simulink model "gm_IP_Core_SS_Switch_and_PWM"  (R2021a)
settings: Solver=VariableStepAuto  StartTime=0.0  StopTime=0.001  RelTol=1e-3
undefined symbols (not defined in the file or in its folder): f_FPGA_clk, T_FPGA_clk
libraries: hdlmdlgenlib x3, hdlsllib x3, simulink x2
(part 2 of 3)

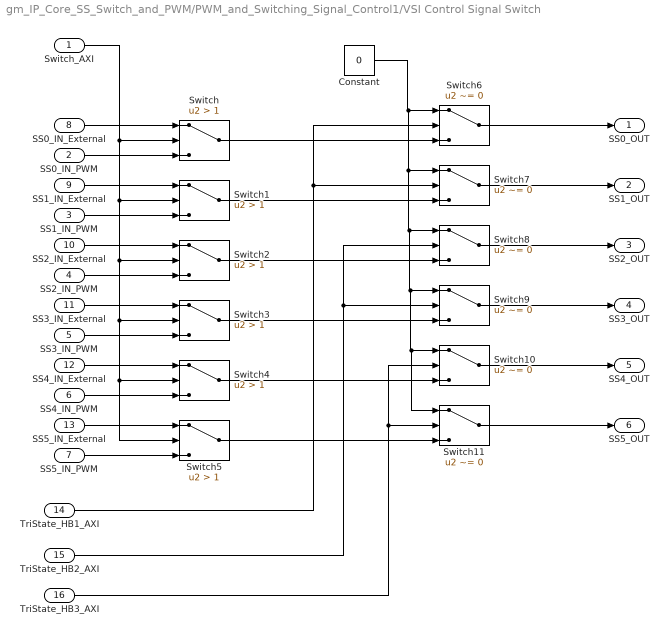
== system gm_IP_Core_SS_Switch_and_PWM/PWM_and_Switching_Signal_Control1/VSI Control Signal Switch ==
  Switch_AXI : Inport
  SS0_IN_PWM : Inport  Port=2
  SS1_IN_PWM : Inport  Port=3
  SS2_IN_PWM : Inport  Port=4
  SS3_IN_PWM : Inport  Port=5
  SS4_IN_PWM : Inport  Port=6
  SS5_IN_PWM : Inport  Port=7
  SS0_IN_External : Inport  Port=8
  SS1_IN_External : Inport  Port=9
  SS2_IN_External : Inport  Port=10
  SS3_IN_External : Inport  Port=11
  SS4_IN_External : Inport  Port=12
  SS5_IN_External : Inport  Port=13
  TriState_HB1_AXI : Inport  Port=14
  TriState_HB2_AXI : Inport  Port=15
  TriState_HB3_AXI : Inport  Port=16
  Constant : Constant  Value=0  OutDataTypeStr=boolean  SampleTime=T_FPGA_clk
  Switch{,1..5} (6 alike) : Switch  Criteria=u2 > Threshold  Threshold=1
  Switch{6..11} (6 alike) : Switch  Criteria=u2 ~= 0  Threshold=1
  SS0_OUT : Outport  VectorParamsAs1DForOutWhenUnconnected=off
  SS1_OUT : Outport  Port=2  VectorParamsAs1DForOutWhenUnconnected=off
  SS2_OUT : Outport  Port=3  VectorParamsAs1DForOutWhenUnconnected=off
  SS3_OUT : Outport  Port=4  VectorParamsAs1DForOutWhenUnconnected=off
  SS4_OUT : Outport  Port=5  VectorParamsAs1DForOutWhenUnconnected=off
  SS5_OUT : Outport  Port=6  VectorParamsAs1DForOutWhenUnconnected=off
  wires:
  Constant/1 -> Switch6/1, Switch7/1, Switch8/1, Switch9/1, Switch10/1, Switch11/1
  Switch6/1 -> SS0_OUT/1
  Switch7/1 -> SS1_OUT/1
  Switch8/1 -> SS2_OUT/1
  Switch9/1 -> SS3_OUT/1
  Switch10/1 -> SS4_OUT/1
  Switch11/1 -> SS5_OUT/1
  TriState_HB1_AXI/1 -> Switch7/2, Switch6/2
  TriState_HB2_AXI/1 -> Switch9/2, Switch8/2
  TriState_HB3_AXI/1 -> Switch11/2, Switch10/2
  SS5_IN_PWM/1 -> Switch5/3
  SS5_IN_External/1 -> Switch5/1
  SS4_IN_PWM/1 -> Switch4/3
  SS4_IN_External/1 -> Switch4/1
  SS3_IN_PWM/1 -> Switch3/3
  SS3_IN_External/1 -> Switch3/1
  SS2_IN_PWM/1 -> Switch2/3
  SS2_IN_External/1 -> Switch2/1
  SS1_IN_PWM/1 -> Switch1/3
  SS1_IN_External/1 -> Switch1/1
  SS0_IN_External/1 -> Switch/1
  SS0_IN_PWM/1 -> Switch/3
  Switch4/1 -> Switch10/3
  Switch1/1 -> Switch7/3
  Switch2/1 -> Switch8/3
  Switch3/1 -> Switch9/3
  Switch/1 -> Switch6/3
  Switch5/1 -> Switch11/3
  Switch_AXI/1 -> Switch/2, Switch1/2, Switch2/2, Switch3/2, Switch5/2, Switch4/2

== system gm_IP_Core_SS_Switch_and_PWM/PWM_and_Switching_Signal_Control/GenPWM/Counter Ctrl ==
  note: scaling triangle amplitude to 100
  hdl_cnt : Inport  OutDataTypeStr=fixdt(0, 20, 0)  PortDimensions=1  SampleTime=1e-08
  f_carrier_kHz : Inport  Port=2  OutDataTypeStr=fixdt(0, 25, 26)  PortDimensions=1  SampleTime=1e-08
  T_carrier_us : Inport  Port=3  OutDataTypeStr=fixdt(0, 25, 0)  PortDimensions=1  SampleTime=1e-08
  Constant1 : Constant  Value=0  OutDataTypeStr=fixdt(0, 20, 0)  SampleTime=1e-08
  Constant11 : Constant  Value=0  OutDataTypeStr=fixdt(0, 20, 0)  SampleTime=1e-08
  Constant12 : Constant  Value=0  OutDataTypeStr=boolean  SampleTime=1e-08
  Constant14 : Constant  OutDataTypeStr=boolean  SampleTime=1e-08
  Delay : Delay  DelayLength=double(1)  InitialCondition=0  SampleTime=1e-08
  Delay6 : Delay  DelayLength=double(1)  InitialCondition=0  SampleTime=1e-08
  Logical Operator : Logic  Operator=OR  AllPortsSameDT=off  OutDataTypeStr=boolean  SampleTime=1e-08
  Product : Product  Inputs=**  OutDataTypeStr=fixdt(0, 18, 17)  SampleTime=1e-08
  Relational Operator1 : RelationalOperator  Operator===  OutDataTypeStr=boolean  SampleTime=1e-08  RndMeth=Nearest
  Relational Operator2 : RelationalOperator  Operator===  OutDataTypeStr=boolean  SampleTime=1e-08  RndMeth=Nearest
  Relational Operator4 : RelationalOperator  OutDataTypeStr=boolean  SampleTime=1e-08  RndMeth=Nearest
  Relational Operator5 : RelationalOperator  Operator=<=  OutDataTypeStr=boolean  SampleTime=1e-08  RndMeth=Nearest
  Switch6 : Switch  Criteria=u2 > Threshold  Threshold=double(0)  OutDataTypeStr=boolean  SampleTime=1e-08
  Switch7 : Switch  Criteria=u2 > Threshold  Threshold=double(0)  OutDataTypeStr=boolean  SampleTime=1e-08
  dir_ctrl : Outport  SampleTime=1e-08  VectorParamsAs1DForOutWhenUnconnected=off
  triangle_sig : Outport  Port=2  SampleTime=1e-08  VectorParamsAs1DForOutWhenUnconnected=off
  Period_CenterMax : Outport  Port=3  SampleTime=1e-08  VectorParamsAs1DForOutWhenUnconnected=off
  Period_CenterMin : Outport  Port=4  SampleTime=1e-08  VectorParamsAs1DForOutWhenUnconnected=off
  wires:
  hdl_cnt/1 -> Relational Operator5/1, Relational Operator4/1, Relational Operator2/1, Relational Operator1/1, Product/1
  f_carrier_kHz/1 -> Delay/1
  T_carrier_us/1 -> Relational Operator4/2, Relational Operator1/2
  Constant1/1 -> Relational Operator2/2
  Constant11/1 -> Relational Operator5/2
  Constant12/1 -> Switch7/1
  Constant14/1 -> Switch7/3
  Delay/1 -> Product/2
  Delay6/1 -> Switch6/3
  Logical Operator/1 -> Switch6/2
  Product/1 -> triangle_sig/1
  Relational Operator1/1 -> Period_CenterMax/1
  Relational Operator2/1 -> Period_CenterMin/1
  Relational Operator4/1 -> Switch7/2, Logical Operator/1
  Relational Operator5/1 -> Logical Operator/2
  Switch6/1 -> Delay6/1, dir_ctrl/1
  Switch7/1 -> Switch6/1

== system gm_IP_Core_SS_Switch_and_PWM/PWM_and_Switching_Signal_Control/GenPWM/LimitPulseWidth ==
  note: Set pulse width between 0-1
  ref_sig : Inport  OutDataTypeStr=fixdt(1, 14, 12)  PortDimensions=1  SampleTime=1e-08
  min_pulse_width : Inport  Port=2  OutDataTypeStr=fixdt(1, 18, 16)  PortDimensions=1  SampleTime=1e-08
  Add : Sum  Inputs=+-  AccumDataTypeStr=fixdt(1, 19, 16)  OutDataTypeStr=fixdt(1, 18, 16)  SampleTime=1e-08
  Constant : Constant  OutDataTypeStr=fixdt(1, 18, 16)  SampleTime=1e-08
  Constant1 : Constant  Value=1.0099945068359375  OutDataTypeStr=fixdt(1, 18, 16)  SampleTime=1e-08
  Constant2 : Constant  Value=0  OutDataTypeStr=fixdt(1, 18, 16)  SampleTime=1e-08
  Logical Operator : Logic  Operator=OR  AllPortsSameDT=off  OutDataTypeStr=boolean  SampleTime=1e-08
  Relational Operator : RelationalOperator  Operator=>  OutDataTypeStr=boolean  SampleTime=1e-08  RndMeth=Nearest
  Relational Operator1 : RelationalOperator  Operator=<  OutDataTypeStr=boolean  SampleTime=1e-08  RndMeth=Nearest
  Saturation : Saturate  UpperLimit="fi(0,1,18,16,\"hex\",\"10000\")"  LowerLimit="fi(0,1,18,16,\"hex\",\"00000\")"  SampleTime=1e-08  OutDataTypeStr=fixdt(1, 18, 16)
  Switch1 : Switch  Criteria=u2 > Threshold  Threshold=double(0)  OutDataTypeStr=fixdt(1, 18, 16)  SampleTime=1e-08
  Switch6 : Switch  Criteria=u2 > Threshold  Threshold=double(0)  OutDataTypeStr=fixdt(1, 18, 16)  SampleTime=1e-08
  ref_sig_limit : Outport  SampleTime=1e-08  VectorParamsAs1DForOutWhenUnconnected=off
  wires:
  Add/1 -> Relational Operator/2
  Constant/1 -> Add/1
  Constant1/1 -> Switch1/3
  Constant2/1 -> Switch1/1
  Logical Operator/1 -> Switch6/2
  Relational Operator/1 -> Logical Operator/1
  Relational Operator1/1 -> Switch1/2, Logical Operator/2
  Saturation/1 -> Relational Operator1/2
  Switch1/1 -> Switch6/1
  Switch6/1 -> ref_sig_limit/1
  ref_sig/1 -> Switch6/3, Relational Operator1/1, Relational Operator/1
  min_pulse_width/1 -> Saturation/1, Add/2

== system gm_IP_Core_SS_Switch_and_PWM/PWM_and_Switching_Signal_Control/GenPWM/LimitPulseWidth1 ==
  note: Set pulse width in percent
  ref_sig : Inport  OutDataTypeStr=fixdt(1, 14, 12)  PortDimensions=1  SampleTime=1e-08
  min_pulse_width : Inport  Port=2  OutDataTypeStr=fixdt(1, 18, 16)  PortDimensions=1  SampleTime=1e-08
  Add : Sum  Inputs=+-  AccumDataTypeStr=fixdt(1, 19, 16)  OutDataTypeStr=fixdt(1, 18, 16)  SampleTime=1e-08
  Constant : Constant  OutDataTypeStr=fixdt(1, 18, 16)  SampleTime=1e-08
  Constant1 : Constant  Value=1.0099945068359375  OutDataTypeStr=fixdt(1, 18, 16)  SampleTime=1e-08
  Constant2 : Constant  Value=0  OutDataTypeStr=fixdt(1, 18, 16)  SampleTime=1e-08
  Logical Operator : Logic  Operator=OR  AllPortsSameDT=off  OutDataTypeStr=boolean  SampleTime=1e-08
  Relational Operator : RelationalOperator  Operator=>  OutDataTypeStr=boolean  SampleTime=1e-08  RndMeth=Nearest
  Relational Operator1 : RelationalOperator  Operator=<  OutDataTypeStr=boolean  SampleTime=1e-08  RndMeth=Nearest
  Saturation : Saturate  UpperLimit="fi(0,1,18,16,\"hex\",\"10000\")"  LowerLimit="fi(0,1,18,16,\"hex\",\"00000\")"  SampleTime=1e-08  OutDataTypeStr=fixdt(1, 18, 16)
  Switch1 : Switch  Criteria=u2 > Threshold  Threshold=double(0)  OutDataTypeStr=fixdt(1, 18, 16)  SampleTime=1e-08
  Switch6 : Switch  Criteria=u2 > Threshold  Threshold=double(0)  OutDataTypeStr=fixdt(1, 18, 16)  SampleTime=1e-08
  ref_sig_limit : Outport  SampleTime=1e-08  VectorParamsAs1DForOutWhenUnconnected=off
  wires:
  Add/1 -> Relational Operator/2
  Constant/1 -> Add/1
  Constant1/1 -> Switch1/3
  Constant2/1 -> Switch1/1
  Logical Operator/1 -> Switch6/2
  Relational Operator/1 -> Logical Operator/1
  Relational Operator1/1 -> Switch1/2, Logical Operator/2
  Saturation/1 -> Relational Operator1/2
  Switch1/1 -> Switch6/1
  Switch6/1 -> ref_sig_limit/1
  ref_sig/1 -> Switch6/3, Relational Operator1/1, Relational Operator/1
  min_pulse_width/1 -> Saturation/1, Add/2

== system gm_IP_Core_SS_Switch_and_PWM/PWM_and_Switching_Signal_Control/GenPWM/LimitPulseWidth2 ==
  note: Set pulse width in percent
  ref_sig : Inport  OutDataTypeStr=fixdt(1, 14, 12)  PortDimensions=1  SampleTime=1e-08
  min_pulse_width : Inport  Port=2  OutDataTypeStr=fixdt(1, 18, 16)  PortDimensions=1  SampleTime=1e-08
  Add : Sum  Inputs=+-  AccumDataTypeStr=fixdt(1, 19, 16)  OutDataTypeStr=fixdt(1, 18, 16)  SampleTime=1e-08
  Constant : Constant  OutDataTypeStr=fixdt(1, 18, 16)  SampleTime=1e-08
  Constant1 : Constant  Value=1.0099945068359375  OutDataTypeStr=fixdt(1, 18, 16)  SampleTime=1e-08
  Constant2 : Constant  Value=0  OutDataTypeStr=fixdt(1, 18, 16)  SampleTime=1e-08
  Logical Operator : Logic  Operator=OR  AllPortsSameDT=off  OutDataTypeStr=boolean  SampleTime=1e-08
  Relational Operator : RelationalOperator  Operator=>  OutDataTypeStr=boolean  SampleTime=1e-08  RndMeth=Nearest
  Relational Operator1 : RelationalOperator  Operator=<  OutDataTypeStr=boolean  SampleTime=1e-08  RndMeth=Nearest
  Saturation : Saturate  UpperLimit="fi(0,1,18,16,\"hex\",\"10000\")"  LowerLimit="fi(0,1,18,16,\"hex\",\"00000\")"  SampleTime=1e-08  OutDataTypeStr=fixdt(1, 18, 16)
  Switch1 : Switch  Criteria=u2 > Threshold  Threshold=double(0)  OutDataTypeStr=fixdt(1, 18, 16)  SampleTime=1e-08
  Switch6 : Switch  Criteria=u2 > Threshold  Threshold=double(0)  OutDataTypeStr=fixdt(1, 18, 16)  SampleTime=1e-08
  ref_sig_limit : Outport  SampleTime=1e-08  VectorParamsAs1DForOutWhenUnconnected=off
  wires:
  Add/1 -> Relational Operator/2
  Constant/1 -> Add/1
  Constant1/1 -> Switch1/3
  Constant2/1 -> Switch1/1
  Logical Operator/1 -> Switch6/2
  Relational Operator/1 -> Logical Operator/1
  Relational Operator1/1 -> Switch1/2, Logical Operator/2
  Saturation/1 -> Relational Operator1/2
  Switch1/1 -> Switch6/1
  Switch6/1 -> ref_sig_limit/1
  ref_sig/1 -> Switch6/3, Relational Operator1/1, Relational Operator/1
  min_pulse_width/1 -> Saturation/1, Add/2

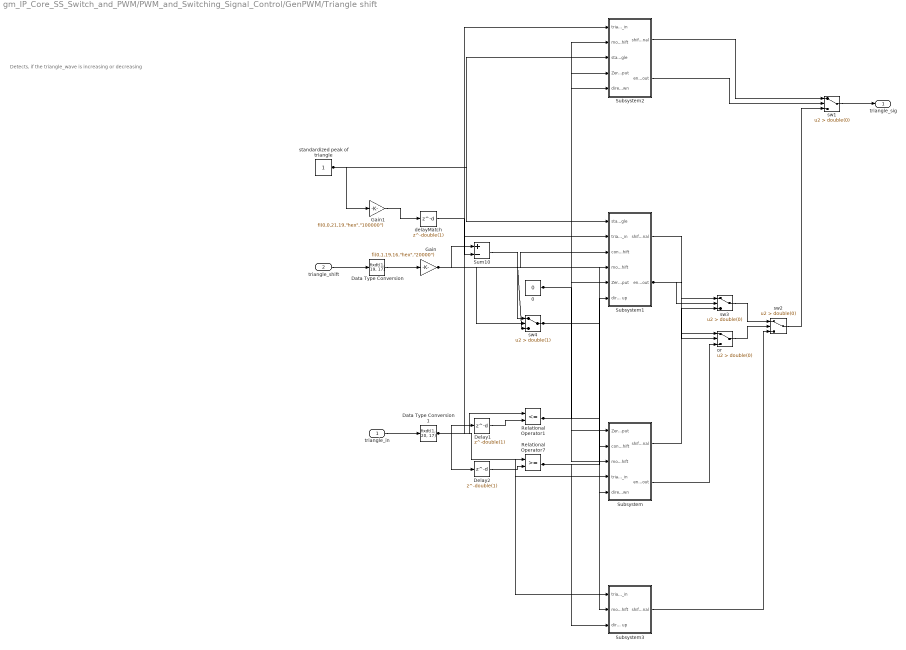
== system gm_IP_Core_SS_Switch_and_PWM/PWM_and_Switching_Signal_Control/GenPWM/Triangle shift ==
  note: Detects, if the triangle_wave is increasing or decreasing
  triangle_in : Inport  OutDataTypeStr=fixdt(0, 18, 17)  PortDimensions=1  SampleTime=1e-08
  triangle_shift : Inport  Port=2  OutDataTypeStr=fixdt(0, 18, 17)  PortDimensions=1  SampleTime=1e-08
  0 : Constant  Value=0  OutDataTypeStr=boolean  SampleTime=1e-08
  Data Type Conversion : DataTypeConversion  OutDataTypeStr=fixdt(1, 19, 17)  SampleTime=1e-08
  Data Type Conversion1 : DataTypeConversion  OutDataTypeStr=fixdt(1, 20, 17)  SampleTime=1e-08
  Delay1 : Delay  DelayLength=double(1)  InitialCondition=0  SampleTime=1e-08
  Delay2 : Delay  DelayLength=double(1)  InitialCondition=0  SampleTime=1e-08
  Gain : Gain  Gain="fi(0,1,19,16,\"hex\",\"20000\")"  ParamDataTypeStr=fixdt(1, 19, 16)  OutDataTypeStr=fixdt(1, 20, 17)  SampleTime=1e-08
  Gain1 : Gain  Gain="fi(0,0,21,19,\"hex\",\"100000\")"  ParamDataTypeStr=fixdt(0, 21, 19)  OutDataTypeStr=fixdt(1, 20, 17)  SampleTime=1e-08
  Relational Operator1 : RelationalOperator  Operator=<=  OutDataTypeStr=boolean  SampleTime=1e-08  RndMeth=Nearest
  Relational Operator7 : RelationalOperator  OutDataTypeStr=boolean  SampleTime=1e-08  RndMeth=Nearest
  Subsystem : Subsystem
  Subsystem1 : Subsystem
  Subsystem2 : Subsystem
  Subsystem3 : Subsystem
  Sum10 : Sum  Inputs=+-  AccumDataTypeStr=fixdt(1, 21, 17)  OutDataTypeStr=fixdt(1, 20, 17)  SampleTime=1e-08
  delayMatch : Delay  DelayLength=double(1)  InitialCondition=0  SampleTime=1e-08
  or : Switch  Criteria=u2 > Threshold  Threshold=double(0)  OutDataTypeStr=boolean  SampleTime=1e-08
  standardized peak of triangle : Constant  OutDataTypeStr=fixdt(0, 21, 17)  SampleTime=1e-08
  sw1 : Switch  Criteria=u2 > Threshold  Threshold=double(0)  OutDataTypeStr=fixdt(1, 18, 16)  SampleTime=1e-08
  sw2 : Switch  Criteria=u2 > Threshold  Threshold=double(0)  OutDataTypeStr=fixdt(1, 21, 17)  SampleTime=1e-08
  sw3 : Switch  Criteria=u2 > Threshold  Threshold=double(0)  OutDataTypeStr=fixdt(1, 21, 17)  SampleTime=1e-08
  sw4 : Switch  Criteria=u2 > Threshold  Threshold=double(1)  OutDataTypeStr=fixdt(1, 20, 17)  SampleTime=1e-08
  triangle_sig : Outport  SampleTime=1e-08  VectorParamsAs1DForOutWhenUnconnected=off
  wires:
  0/1 -> Subsystem2/4(Zero_input), Subsystem1/5(Zero_input), Subsystem/1(Zero_input)
  Data Type Conversion/1 -> Gain/1
  Data Type Conversion1/1 -> Relational Operator7/1, Relational Operator1/1, Delay2/1, Delay1/1, Subsystem3/1(triangle_in), Subsystem2/1(triangle_in), Subsystem/4(triangle_in), Subsystem1/2(triangle_in)
  Delay1/1 -> Relational Operator1/2
  Delay2/1 -> Relational Operator7/2
  Gain/1 -> sw4/3, sw4/2, Sum10/1, Subsystem/2(converted triangle_shift), Subsystem1/3(converted triangle_shift)
  delayMatch/1 -> Sum10/2
  Relational Operator1/1 -> Subsystem/5(direction down), Subsystem2/5(direction down)
  Relational Operator7/1 -> Subsystem1/6(direction up), Subsystem3/3(direction up)
  Subsystem/1(shifted triangle_in signal) -> sw3/3
  Subsystem/2(enable_out) -> or/3
  Subsystem1/1(shifted triangle_in signal) -> sw3/1
  Subsystem1/2(enable_out) -> sw3/2, or/2, or/1
  Subsystem2/1(shifted triangle_in signal) -> sw1/1
  Subsystem2/2(enable_out) -> sw1/2
  Subsystem3/1(shifted triangle_in signal) -> sw2/3
  Sum10/1 -> sw4/1
  or/1 -> sw2/2
  standardized peak of triangle/1 -> Gain1/1, Subsystem2/3(standardized peak of triangle), Subsystem1/1(standardized peak of triangle)
  sw1/1 -> triangle_sig/1
  sw2/1 -> sw1/3
  sw3/1 -> sw2/1
  sw4/1 -> Subsystem3/2(modified triangle_shift), Subsystem/3(modified triangle_shift), Subsystem1/4(modified triangle_shift), Subsystem2/2(modified triangle_shift)
  triangle_in/1 -> Data Type Conversion1/1
  triangle_shift/1 -> Data Type Conversion/1
  Gain1/1 -> delayMatch/1

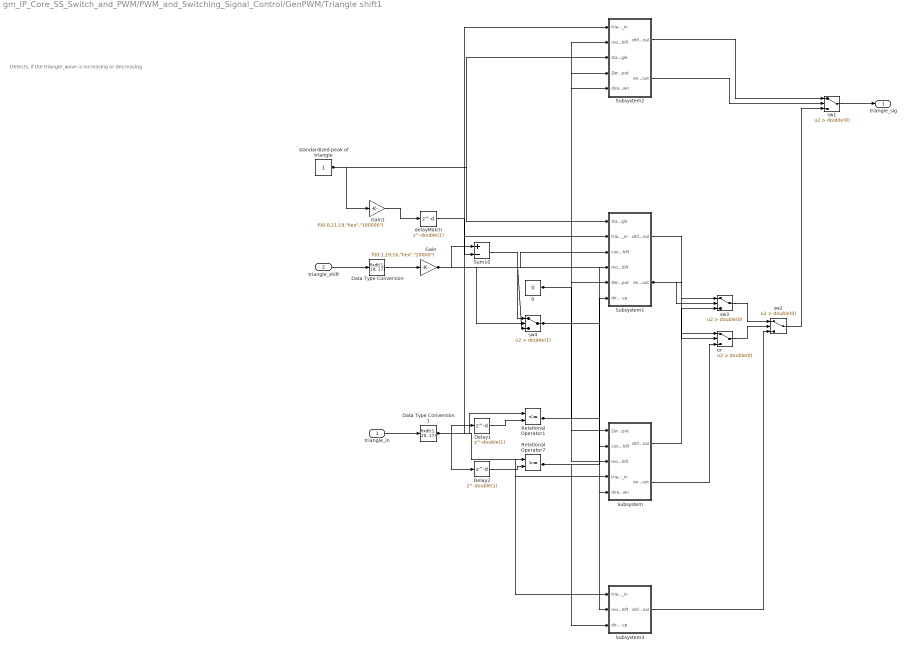
== system gm_IP_Core_SS_Switch_and_PWM/PWM_and_Switching_Signal_Control/GenPWM/Triangle shift1 ==
  note: Detects, if the triangle_wave is increasing or decreasing
  triangle_in : Inport  OutDataTypeStr=fixdt(0, 18, 17)  PortDimensions=1  SampleTime=1e-08
  triangle_shift : Inport  Port=2  OutDataTypeStr=fixdt(0, 18, 17)  PortDimensions=1  SampleTime=1e-08
  0 : Constant  Value=0  OutDataTypeStr=boolean  SampleTime=1e-08
  Data Type Conversion : DataTypeConversion  OutDataTypeStr=fixdt(1, 19, 17)  SampleTime=1e-08
  Data Type Conversion1 : DataTypeConversion  OutDataTypeStr=fixdt(1, 20, 17)  SampleTime=1e-08
  Delay1 : Delay  DelayLength=double(1)  InitialCondition=0  SampleTime=1e-08
  Delay2 : Delay  DelayLength=double(1)  InitialCondition=0  SampleTime=1e-08
  Gain : Gain  Gain="fi(0,1,19,16,\"hex\",\"20000\")"  ParamDataTypeStr=fixdt(1, 19, 16)  OutDataTypeStr=fixdt(1, 20, 17)  SampleTime=1e-08
  Gain1 : Gain  Gain="fi(0,0,21,19,\"hex\",\"100000\")"  ParamDataTypeStr=fixdt(0, 21, 19)  OutDataTypeStr=fixdt(1, 20, 17)  SampleTime=1e-08
  Relational Operator1 : RelationalOperator  Operator=<=  OutDataTypeStr=boolean  SampleTime=1e-08  RndMeth=Nearest
  Relational Operator7 : RelationalOperator  OutDataTypeStr=boolean  SampleTime=1e-08  RndMeth=Nearest
  Subsystem : Subsystem
  Subsystem1 : Subsystem
  Subsystem2 : Subsystem
  Subsystem3 : Subsystem
  Sum10 : Sum  Inputs=+-  AccumDataTypeStr=fixdt(1, 21, 17)  OutDataTypeStr=fixdt(1, 20, 17)  SampleTime=1e-08
  delayMatch : Delay  DelayLength=double(1)  InitialCondition=0  SampleTime=1e-08
  or : Switch  Criteria=u2 > Threshold  Threshold=double(0)  OutDataTypeStr=boolean  SampleTime=1e-08
  standardized peak of triangle : Constant  OutDataTypeStr=fixdt(0, 21, 17)  SampleTime=1e-08
  sw1 : Switch  Criteria=u2 > Threshold  Threshold=double(0)  OutDataTypeStr=fixdt(1, 18, 16)  SampleTime=1e-08
  sw2 : Switch  Criteria=u2 > Threshold  Threshold=double(0)  OutDataTypeStr=fixdt(1, 21, 17)  SampleTime=1e-08
  sw3 : Switch  Criteria=u2 > Threshold  Threshold=double(0)  OutDataTypeStr=fixdt(1, 21, 17)  SampleTime=1e-08
  sw4 : Switch  Criteria=u2 > Threshold  Threshold=double(1)  OutDataTypeStr=fixdt(1, 20, 17)  SampleTime=1e-08
  triangle_sig : Outport  SampleTime=1e-08  VectorParamsAs1DForOutWhenUnconnected=off
  wires:
  0/1 -> Subsystem2/4(Zero_input), Subsystem1/5(Zero_input), Subsystem/1(Zero_input)
  Data Type Conversion/1 -> Gain/1
  Data Type Conversion1/1 -> Relational Operator7/1, Relational Operator1/1, Delay2/1, Delay1/1, Subsystem3/1(triangle_in), Subsystem2/1(triangle_in), Subsystem/4(triangle_in), Subsystem1/2(triangle_in)
  Delay1/1 -> Relational Operator1/2
  Delay2/1 -> Relational Operator7/2
  Gain/1 -> sw4/3, sw4/2, Sum10/1, Subsystem/2(converted triangle_shift), Subsystem1/3(converted triangle_shift)
  delayMatch/1 -> Sum10/2
  Relational Operator1/1 -> Subsystem/5(direction down), Subsystem2/5(direction down)
  Relational Operator7/1 -> Subsystem1/6(direction up), Subsystem3/3(direction up)
  Subsystem/1(shifted triangle_in signal) -> sw3/3
  Subsystem/2(enable_out) -> or/3
  Subsystem1/1(shifted triangle_in signal) -> sw3/1
  Subsystem1/2(enable_out) -> sw3/2, or/2, or/1
  Subsystem2/1(shifted triangle_in signal) -> sw1/1
  Subsystem2/2(enable_out) -> sw1/2
  Subsystem3/1(shifted triangle_in signal) -> sw2/3
  Sum10/1 -> sw4/1
  or/1 -> sw2/2
  standardized peak of triangle/1 -> Gain1/1, Subsystem2/3(standardized peak of triangle), Subsystem1/1(standardized peak of triangle)
  sw1/1 -> triangle_sig/1
  sw2/1 -> sw1/3
  sw3/1 -> sw2/1
  sw4/1 -> Subsystem3/2(modified triangle_shift), Subsystem/3(modified triangle_shift), Subsystem1/4(modified triangle_shift), Subsystem2/2(modified triangle_shift)
  triangle_in/1 -> Data Type Conversion1/1
  triangle_shift/1 -> Data Type Conversion/1
  Gain1/1 -> delayMatch/1

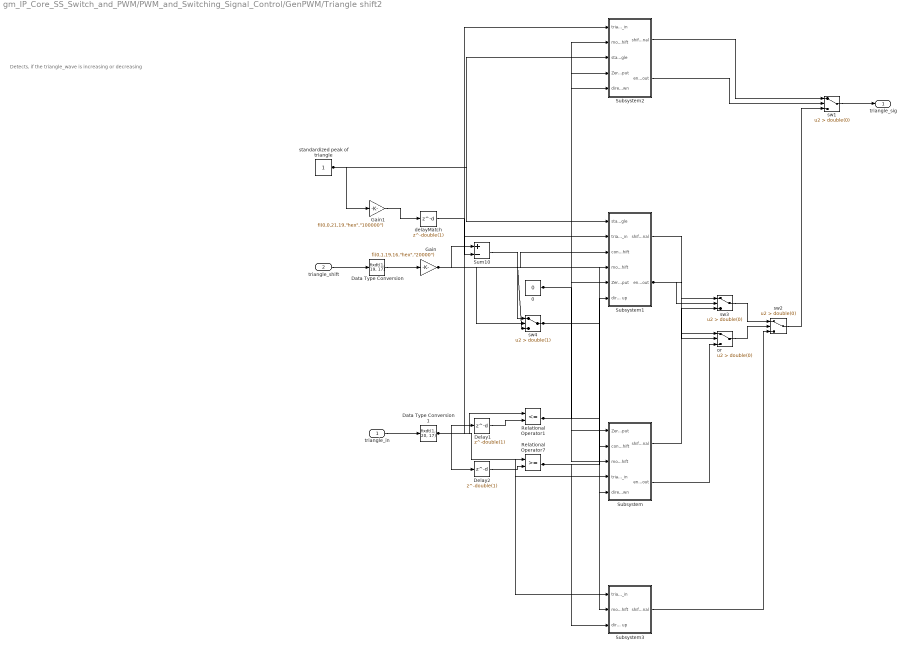
== system gm_IP_Core_SS_Switch_and_PWM/PWM_and_Switching_Signal_Control/GenPWM/Triangle shift2 ==
  note: Detects, if the triangle_wave is increasing or decreasing
  triangle_in : Inport  OutDataTypeStr=fixdt(0, 18, 17)  PortDimensions=1  SampleTime=1e-08
  triangle_shift : Inport  Port=2  OutDataTypeStr=fixdt(0, 18, 17)  PortDimensions=1  SampleTime=1e-08
  0 : Constant  Value=0  OutDataTypeStr=boolean  SampleTime=1e-08
  Data Type Conversion : DataTypeConversion  OutDataTypeStr=fixdt(1, 19, 17)  SampleTime=1e-08
  Data Type Conversion1 : DataTypeConversion  OutDataTypeStr=fixdt(1, 20, 17)  SampleTime=1e-08
  Delay1 : Delay  DelayLength=double(1)  InitialCondition=0  SampleTime=1e-08
  Delay2 : Delay  DelayLength=double(1)  InitialCondition=0  SampleTime=1e-08
  Gain : Gain  Gain="fi(0,1,19,16,\"hex\",\"20000\")"  ParamDataTypeStr=fixdt(1, 19, 16)  OutDataTypeStr=fixdt(1, 20, 17)  SampleTime=1e-08
  Gain1 : Gain  Gain="fi(0,0,21,19,\"hex\",\"100000\")"  ParamDataTypeStr=fixdt(0, 21, 19)  OutDataTypeStr=fixdt(1, 20, 17)  SampleTime=1e-08
  Relational Operator1 : RelationalOperator  Operator=<=  OutDataTypeStr=boolean  SampleTime=1e-08  RndMeth=Nearest
  Relational Operator7 : RelationalOperator  OutDataTypeStr=boolean  SampleTime=1e-08  RndMeth=Nearest
  Subsystem : Subsystem
  Subsystem1 : Subsystem
  Subsystem2 : Subsystem
  Subsystem3 : Subsystem
  Sum10 : Sum  Inputs=+-  AccumDataTypeStr=fixdt(1, 21, 17)  OutDataTypeStr=fixdt(1, 20, 17)  SampleTime=1e-08
  delayMatch : Delay  DelayLength=double(1)  InitialCondition=0  SampleTime=1e-08
  or : Switch  Criteria=u2 > Threshold  Threshold=double(0)  OutDataTypeStr=boolean  SampleTime=1e-08
  standardized peak of triangle : Constant  OutDataTypeStr=fixdt(0, 21, 17)  SampleTime=1e-08
  sw1 : Switch  Criteria=u2 > Threshold  Threshold=double(0)  OutDataTypeStr=fixdt(1, 18, 16)  SampleTime=1e-08
  sw2 : Switch  Criteria=u2 > Threshold  Threshold=double(0)  OutDataTypeStr=fixdt(1, 21, 17)  SampleTime=1e-08
  sw3 : Switch  Criteria=u2 > Threshold  Threshold=double(0)  OutDataTypeStr=fixdt(1, 21, 17)  SampleTime=1e-08
  sw4 : Switch  Criteria=u2 > Threshold  Threshold=double(1)  OutDataTypeStr=fixdt(1, 20, 17)  SampleTime=1e-08
  triangle_sig : Outport  SampleTime=1e-08  VectorParamsAs1DForOutWhenUnconnected=off
  wires:
  0/1 -> Subsystem2/4(Zero_input), Subsystem1/5(Zero_input), Subsystem/1(Zero_input)
  Data Type Conversion/1 -> Gain/1
  Data Type Conversion1/1 -> Relational Operator7/1, Relational Operator1/1, Delay2/1, Delay1/1, Subsystem3/1(triangle_in), Subsystem2/1(triangle_in), Subsystem/4(triangle_in), Subsystem1/2(triangle_in)
  Delay1/1 -> Relational Operator1/2
  Delay2/1 -> Relational Operator7/2
  Gain/1 -> sw4/3, sw4/2, Sum10/1, Subsystem/2(converted triangle_shift), Subsystem1/3(converted triangle_shift)
  delayMatch/1 -> Sum10/2
  Relational Operator1/1 -> Subsystem/5(direction down), Subsystem2/5(direction down)
  Relational Operator7/1 -> Subsystem1/6(direction up), Subsystem3/3(direction up)
  Subsystem/1(shifted triangle_in signal) -> sw3/3
  Subsystem/2(enable_out) -> or/3
  Subsystem1/1(shifted triangle_in signal) -> sw3/1
  Subsystem1/2(enable_out) -> sw3/2, or/2, or/1
  Subsystem2/1(shifted triangle_in signal) -> sw1/1
  Subsystem2/2(enable_out) -> sw1/2
  Subsystem3/1(shifted triangle_in signal) -> sw2/3
  Sum10/1 -> sw4/1
  or/1 -> sw2/2
  standardized peak of triangle/1 -> Gain1/1, Subsystem2/3(standardized peak of triangle), Subsystem1/1(standardized peak of triangle)
  sw1/1 -> triangle_sig/1
  sw2/1 -> sw1/3
  sw3/1 -> sw2/1
  sw4/1 -> Subsystem3/2(modified triangle_shift), Subsystem/3(modified triangle_shift), Subsystem1/4(modified triangle_shift), Subsystem2/2(modified triangle_shift)
  triangle_in/1 -> Data Type Conversion1/1
  triangle_shift/1 -> Data Type Conversion/1
  Gain1/1 -> delayMatch/1

== system gm_IP_Core_SS_Switch_and_PWM/PWM_and_Switching_Signal_Control1/GenPWM/Counter Ctrl ==
  note: scaling triangle amplitude to 100
  note: if (hdl_cnt >= step_cnt)
      | 	dir_ctrl = true;
      | else if (hdl_cnt <= 0)
      | 	dir_ctrl = false;
      | else
      | 	dir_ctrl = dir_ctrl;
  hdl_cnt : Inport
  f_carrier_kHz : Inport  Port=2
  T_carrier_us : Inport  Port=3
  Constant1 : Constant  Value=0  OutDataTypeStr=fixdt(0,20,0)  SampleTime=T_FPGA_clk
  Constant11 : Constant  Value=0  OutDataTypeStr=fixdt(0,20,0)  SampleTime=T_FPGA_clk
  Constant12 : Constant  Value=false  SampleTime=T_FPGA_clk
  Constant14 : Constant  Value=true  SampleTime=T_FPGA_clk
  Delay : Delay  DelayLength=1
  Delay6 : Delay  DelayLength=1
  Logical Operator : Logic  Operator=OR  AllPortsSameDT=off  OutDataTypeStr=boolean
  Product : Product  OutDataTypeStr=fixdt(0,18,17)
  Relational Operator1 : RelationalOperator  Operator===  OutDataTypeStr=boolean  RndMeth=Nearest
  Relational Operator2 : RelationalOperator  Operator===  OutDataTypeStr=boolean  RndMeth=Nearest
  Relational Operator4 : RelationalOperator  OutDataTypeStr=boolean  RndMeth=Nearest
  Relational Operator5 : RelationalOperator  Operator=<=  OutDataTypeStr=boolean  RndMeth=Nearest
  Scope9 : Scope  NumInputPorts=2
  Switch6 : Switch  Criteria=u2 > Threshold
  Switch7 : Switch  Criteria=u2 > Threshold
  dir_ctrl : Outport  VectorParamsAs1DForOutWhenUnconnected=off
  triangle_sig : Outport  Port=2  VectorParamsAs1DForOutWhenUnconnected=off
  Period_CenterMax : Outport  Port=3  VectorParamsAs1DForOutWhenUnconnected=off
  Period_CenterMin : Outport  Port=4  VectorParamsAs1DForOutWhenUnconnected=off
  wires:
  Product/1 -> triangle_sig/1
  Constant1/1 -> Relational Operator2/2
  Relational Operator2/1 -> Period_CenterMin/1
  Relational Operator1/1 -> Period_CenterMax/1
  Delay/1 -> Product/2, Scope9/2
  f_carrier_kHz/1 -> Delay/1
  T_carrier_us/1 -> Relational Operator1/2, Relational Operator4/2
  Delay6/1 -> Switch6/3
  Constant14/1 -> Switch7/3
  Constant12/1 -> Switch7/1
  Switch7/1 -> Switch6/1
  Logical Operator/1 -> Switch6/2
  Constant11/1 -> Relational Operator5/2
  Relational Operator5/1 -> Logical Operator/2
  Relational Operator4/1 -> Logical Operator/1, Switch7/2
  Switch6/1 -> dir_ctrl/1, Delay6/1
  hdl_cnt/1 -> Scope9/1, Product/1, Relational Operator4/1, Relational Operator5/1, Relational Operator1/1, Relational Operator2/1

== system gm_IP_Core_SS_Switch_and_PWM/PWM_and_Switching_Signal_Control1/GenPWM/LimitPulseWidth ==
  note: Set pulse width between 0-1
  ref_sig : Inport
  min_pulse_width : Inport  Port=2
  Add : Sum  Inputs=+-  OutDataTypeStr=Inherit: Same as first input
  Constant : Constant  OutDataTypeStr=fixdt(1,18,16)  SampleTime=T_FPGA_clk
  Constant1 : Constant  Value=1.01  OutDataTypeStr=fixdt(1,18,16)  SampleTime=T_FPGA_clk
  Constant2 : Constant  Value=0  OutDataTypeStr=fixdt(1,18,16)  SampleTime=T_FPGA_clk
  Logical Operator : Logic  Operator=OR  AllPortsSameDT=off  OutDataTypeStr=boolean
  Relational Operator : RelationalOperator  Operator=>  OutDataTypeStr=boolean  RndMeth=Nearest
  Relational Operator1 : RelationalOperator  Operator=<  OutDataTypeStr=boolean  RndMeth=Nearest
  Saturation : Saturate  UpperLimit=1  LowerLimit=0  OutDataTypeStr=fixdt(1,18,16)
  Switch1 : Switch  Criteria=u2 > Threshold
  Switch6 : Switch  Criteria=u2 > Threshold
  ref_sig_limit : Outport  VectorParamsAs1DForOutWhenUnconnected=off
  wires:
  Saturation/1 -> Relational Operator1/2
  Switch6/1 -> ref_sig_limit/1
  Constant2/1 -> Switch1/1
  Switch1/1 -> Switch6/1
  Constant1/1 -> Switch1/3
  Logical Operator/1 -> Switch6/2
  Relational Operator1/1 -> Switch1/2, Logical Operator/2
  Relational Operator/1 -> Logical Operator/1
  ref_sig/1 -> Relational Operator1/1, Relational Operator/1, Switch6/3
  Add/1 -> Relational Operator/2
  min_pulse_width/1 -> Saturation/1, Add/2
  Constant/1 -> Add/1

== system gm_IP_Core_SS_Switch_and_PWM/PWM_and_Switching_Signal_Control1/GenPWM/LimitPulseWidth1 ==
  note: Set pulse width in percent
  ref_sig : Inport
  min_pulse_width : Inport  Port=2
  Add : Sum  Inputs=+-  OutDataTypeStr=Inherit: Same as first input
  Constant : Constant  OutDataTypeStr=fixdt(1,18,16)  SampleTime=T_FPGA_clk
  Constant1 : Constant  Value=1.01  OutDataTypeStr=fixdt(1,18,16)  SampleTime=T_FPGA_clk
  Constant2 : Constant  Value=0  OutDataTypeStr=fixdt(1,18,16)  SampleTime=T_FPGA_clk
  Logical Operator : Logic  Operator=OR  AllPortsSameDT=off  OutDataTypeStr=boolean
  Relational Operator : RelationalOperator  Operator=>  OutDataTypeStr=boolean  RndMeth=Nearest
  Relational Operator1 : RelationalOperator  Operator=<  OutDataTypeStr=boolean  RndMeth=Nearest
  Saturation : Saturate  UpperLimit=1  LowerLimit=0  OutDataTypeStr=fixdt(1,18,16)
  Switch1 : Switch  Criteria=u2 > Threshold
  Switch6 : Switch  Criteria=u2 > Threshold
  ref_sig_limit : Outport  VectorParamsAs1DForOutWhenUnconnected=off
  wires:
  Saturation/1 -> Relational Operator1/2
  Switch6/1 -> ref_sig_limit/1
  Constant2/1 -> Switch1/1
  Switch1/1 -> Switch6/1
  Constant1/1 -> Switch1/3
  Logical Operator/1 -> Switch6/2
  Relational Operator1/1 -> Switch1/2, Logical Operator/2
  Relational Operator/1 -> Logical Operator/1
  ref_sig/1 -> Relational Operator1/1, Relational Operator/1, Switch6/3
  Add/1 -> Relational Operator/2
  min_pulse_width/1 -> Saturation/1, Add/2
  Constant/1 -> Add/1

== system gm_IP_Core_SS_Switch_and_PWM/PWM_and_Switching_Signal_Control1/GenPWM/LimitPulseWidth2 ==
  note: Set pulse width in percent
  ref_sig : Inport
  min_pulse_width : Inport  Port=2
  Add : Sum  Inputs=+-  OutDataTypeStr=Inherit: Same as first input
  Constant : Constant  OutDataTypeStr=fixdt(1,18,16)  SampleTime=T_FPGA_clk
  Constant1 : Constant  Value=1.01  OutDataTypeStr=fixdt(1,18,16)  SampleTime=T_FPGA_clk
  Constant2 : Constant  Value=0  OutDataTypeStr=fixdt(1,18,16)  SampleTime=T_FPGA_clk
  Logical Operator : Logic  Operator=OR  AllPortsSameDT=off  OutDataTypeStr=boolean
  Relational Operator : RelationalOperator  Operator=>  OutDataTypeStr=boolean  RndMeth=Nearest
  Relational Operator1 : RelationalOperator  Operator=<  OutDataTypeStr=boolean  RndMeth=Nearest
  Saturation : Saturate  UpperLimit=1  LowerLimit=0  OutDataTypeStr=fixdt(1,18,16)
  Switch1 : Switch  Criteria=u2 > Threshold
  Switch6 : Switch  Criteria=u2 > Threshold
  ref_sig_limit : Outport  VectorParamsAs1DForOutWhenUnconnected=off
  wires:
  Saturation/1 -> Relational Operator1/2
  Switch6/1 -> ref_sig_limit/1
  Constant2/1 -> Switch1/1
  Switch1/1 -> Switch6/1
  Constant1/1 -> Switch1/3
  Logical Operator/1 -> Switch6/2
  Relational Operator1/1 -> Switch1/2, Logical Operator/2
  Relational Operator/1 -> Logical Operator/1
  ref_sig/1 -> Relational Operator1/1, Relational Operator/1, Switch6/3
  Add/1 -> Relational Operator/2
  min_pulse_width/1 -> Saturation/1, Add/2
  Constant/1 -> Add/1

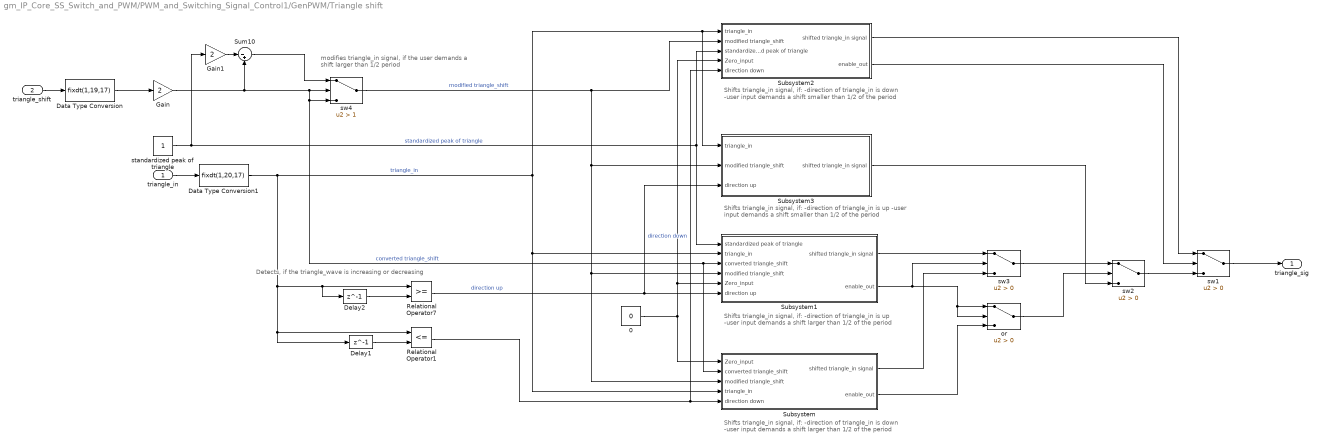
== system gm_IP_Core_SS_Switch_and_PWM/PWM_and_Switching_Signal_Control1/GenPWM/Triangle shift ==
  note: Shifts triangle_in signal, if:
      | -direction of triangle_in is down
      | -user input demands a shift smaller than 1/2 of the period
  note: Shifts triangle_in signal, if:
      | -direction of triangle_in is up
      | -user input demands a shift smaller than 1/2 of the period
  note: Shifts triangle_in signal, if:
      | -direction of triangle_in is up
      | -user input demands a shift larger than 1/2 of the period
  note: Shifts triangle_in signal, if:
      | -direction of triangle_in is down
      | -user input demands a shift larger than 1/2 of the period
  note: Detects, if the triangle_wave is increasing or decreasing
  note: modifies triangle_in signal,
      | if the user demands a shift larger than 1/2 period
  triangle_in : Inport
  triangle_shift : Inport  Port=2
  0 : Constant  Value=0  OutDataTypeStr=boolean  SampleTime=T_FPGA_clk
  Data Type Conversion : DataTypeConversion  OutDataTypeStr=fixdt(1,19,17)
  Data Type Conversion1 : DataTypeConversion  OutDataTypeStr=fixdt(1,20,17)
  Delay1 : Delay  DelayLength=1
  Delay2 : Delay  DelayLength=1
  Gain : Gain  Gain=2  OutDataTypeStr=fixdt(1,20,17)
  Gain1 : Gain  Gain=2  OutDataTypeStr=fixdt(1,20,17)
  Relational Operator1 : RelationalOperator  Operator=<=  OutDataTypeStr=boolean  RndMeth=Nearest
  Relational Operator7 : RelationalOperator  OutDataTypeStr=boolean  RndMeth=Nearest
  Subsystem : Subsystem
  Subsystem1 : Subsystem
  Subsystem2 : Subsystem
  Subsystem3 : Subsystem
  Sum10 : Sum  Inputs=|-+  OutDataTypeStr=fixdt(1,20,17)
  or : Switch  Criteria=u2 > Threshold
  standardized peak of triangle : Constant  OutDataTypeStr=fixdt(0,21,17)  SampleTime=T_FPGA_clk
  sw1 : Switch  Criteria=u2 > Threshold  OutDataTypeStr=fixdt(1,18,16)
  sw2 : Switch  Criteria=u2 > Threshold
  sw3 : Switch  Criteria=u2 > Threshold
  sw4 : Switch  Criteria=u2 > Threshold  Threshold=1  OutDataTypeStr=fixdt(1,20,17)
  triangle_sig : Outport  VectorParamsAs1DForOutWhenUnconnected=off
  wires:
  Subsystem3/1(shifted triangle_in signal) -> sw2/3
  Subsystem2/2(enable_out) -> sw1/2
  Subsystem2/1(shifted triangle_in signal) -> sw1/1
  Subsystem1/1(shifted triangle_in signal) -> sw3/1
  Subsystem1/2(enable_out) -> sw3/2, or/1, or/2
  Subsystem/2(enable_out) -> or/3
  Subsystem/1(shifted triangle_in signal) -> sw3/3
  0/1 -> Subsystem/1(Zero_input), Subsystem1/5(Zero_input), Subsystem2/4(Zero_input)
  Delay1/1 -> Relational Operator1/2
  Relational Operator1/1 -> Subsystem2/5(direction down), Subsystem/5(direction down)  "direction down"
  triangle_in/1 -> Data Type Conversion1/1
  Data Type Conversion/1 -> Gain/1
  sw2/1 -> sw1/3
  Gain1/1 -> Sum10/1
  triangle_shift/1 -> Data Type Conversion/1
  standardized peak of triangle/1 -> Gain1/1, Subsystem1/1(standardized peak of triangle), Subsystem2/3(standardized peak of triangle)  "standardized peak of triangle"
  sw1/1 -> triangle_sig/1
  Sum10/1 -> sw4/1
  Gain/1 -> sw4/2, sw4/3, Subsystem1/3(converted triangle_shift), Subsystem/2(converted triangle_shift), Sum10/2  "converted triangle_shift"
  sw4/1 -> Subsystem2/2(modified triangle_shift), Subsystem1/4(modified triangle_shift), Subsystem/3(modified triangle_shift), Subsystem3/2(modified triangle_shift)  "modified triangle_shift"
  or/1 -> sw2/2
  Relational Operator7/1 -> Subsystem3/3(direction up), Subsystem1/6(direction up)  "direction up"
  sw3/1 -> sw2/1
  Data Type Conversion1/1 -> Relational Operator7/1, Delay2/1, Delay1/1, Relational Operator1/1, Subsystem1/2(triangle_in), Subsystem/4(triangle_in), Subsystem2/1(triangle_in), Subsystem3/1(triangle_in)  "triangle_in"
  Delay2/1 -> Relational Operator7/2

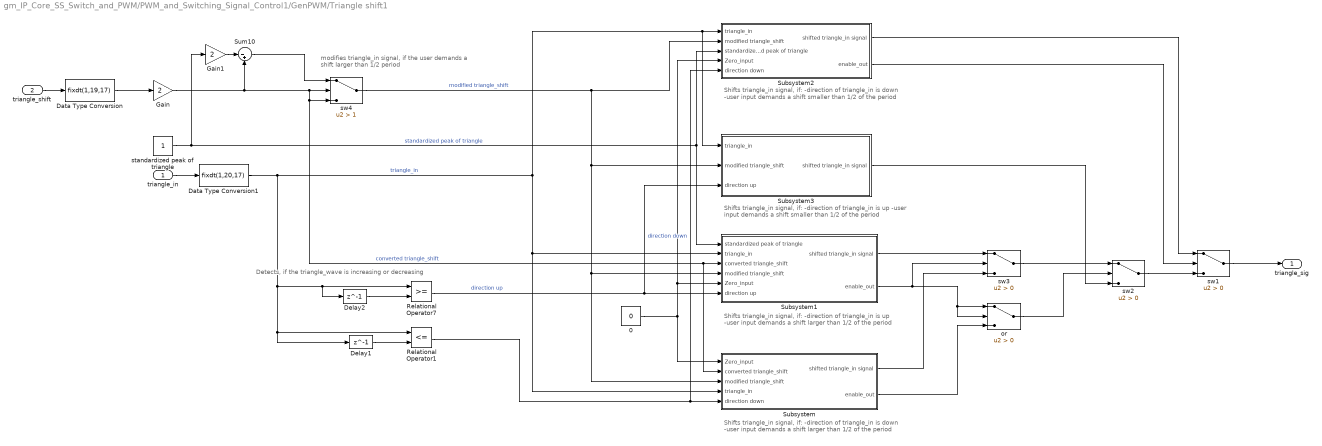
== system gm_IP_Core_SS_Switch_and_PWM/PWM_and_Switching_Signal_Control1/GenPWM/Triangle shift1 ==
  note: Shifts triangle_in signal, if:
      | -direction of triangle_in is down
      | -user input demands a shift smaller than 1/2 of the period
  note: Shifts triangle_in signal, if:
      | -direction of triangle_in is up
      | -user input demands a shift smaller than 1/2 of the period
  note: Shifts triangle_in signal, if:
      | -direction of triangle_in is up
      | -user input demands a shift larger than 1/2 of the period
  note: Shifts triangle_in signal, if:
      | -direction of triangle_in is down
      | -user input demands a shift larger than 1/2 of the period
  note: Detects, if the triangle_wave is increasing or decreasing
  note: modifies triangle_in signal,
      | if the user demands a shift larger than 1/2 period
  triangle_in : Inport
  triangle_shift : Inport  Port=2
  0 : Constant  Value=0  OutDataTypeStr=boolean  SampleTime=T_FPGA_clk
  Data Type Conversion : DataTypeConversion  OutDataTypeStr=fixdt(1,19,17)
  Data Type Conversion1 : DataTypeConversion  OutDataTypeStr=fixdt(1,20,17)
  Delay1 : Delay  DelayLength=1
  Delay2 : Delay  DelayLength=1
  Gain : Gain  Gain=2  OutDataTypeStr=fixdt(1,20,17)
  Gain1 : Gain  Gain=2  OutDataTypeStr=fixdt(1,20,17)
  Relational Operator1 : RelationalOperator  Operator=<=  OutDataTypeStr=boolean  RndMeth=Nearest
  Relational Operator7 : RelationalOperator  OutDataTypeStr=boolean  RndMeth=Nearest
  Subsystem : Subsystem
  Subsystem1 : Subsystem
  Subsystem2 : Subsystem
  Subsystem3 : Subsystem
  Sum10 : Sum  Inputs=|-+  OutDataTypeStr=fixdt(1,20,17)
  or : Switch  Criteria=u2 > Threshold
  standardized peak of triangle : Constant  OutDataTypeStr=fixdt(0,21,17)  SampleTime=T_FPGA_clk
  sw1 : Switch  Criteria=u2 > Threshold  OutDataTypeStr=fixdt(1,18,16)
  sw2 : Switch  Criteria=u2 > Threshold
  sw3 : Switch  Criteria=u2 > Threshold
  sw4 : Switch  Criteria=u2 > Threshold  Threshold=1  OutDataTypeStr=fixdt(1,20,17)
  triangle_sig : Outport  VectorParamsAs1DForOutWhenUnconnected=off
  wires:
  Subsystem3/1(shifted triangle_in signal) -> sw2/3
  Subsystem2/2(enable_out) -> sw1/2
  Subsystem2/1(shifted triangle_in signal) -> sw1/1
  Subsystem1/1(shifted triangle_in signal) -> sw3/1
  Subsystem1/2(enable_out) -> sw3/2, or/1, or/2
  Subsystem/2(enable_out) -> or/3
  Subsystem/1(shifted triangle_in signal) -> sw3/3
  0/1 -> Subsystem/1(Zero_input), Subsystem1/5(Zero_input), Subsystem2/4(Zero_input)
  Delay1/1 -> Relational Operator1/2
  Relational Operator1/1 -> Subsystem2/5(direction down), Subsystem/5(direction down)  "direction down"
  triangle_in/1 -> Data Type Conversion1/1
  Data Type Conversion/1 -> Gain/1
  sw2/1 -> sw1/3
  Gain1/1 -> Sum10/1
  triangle_shift/1 -> Data Type Conversion/1
  standardized peak of triangle/1 -> Gain1/1, Subsystem1/1(standardized peak of triangle), Subsystem2/3(standardized peak of triangle)  "standardized peak of triangle"
  sw1/1 -> triangle_sig/1
  Sum10/1 -> sw4/1
  Gain/1 -> sw4/2, sw4/3, Subsystem1/3(converted triangle_shift), Subsystem/2(converted triangle_shift), Sum10/2  "converted triangle_shift"
  sw4/1 -> Subsystem2/2(modified triangle_shift), Subsystem1/4(modified triangle_shift), Subsystem/3(modified triangle_shift), Subsystem3/2(modified triangle_shift)  "modified triangle_shift"
  or/1 -> sw2/2
  Relational Operator7/1 -> Subsystem3/3(direction up), Subsystem1/6(direction up)  "direction up"
  sw3/1 -> sw2/1
  Data Type Conversion1/1 -> Relational Operator7/1, Delay2/1, Delay1/1, Relational Operator1/1, Subsystem1/2(triangle_in), Subsystem/4(triangle_in), Subsystem2/1(triangle_in), Subsystem3/1(triangle_in)  "triangle_in"
  Delay2/1 -> Relational Operator7/2

== system gm_IP_Core_SS_Switch_and_PWM/PWM_and_Switching_Signal_Control1/GenPWM/Triangle shift2 ==
  note: Shifts triangle_in signal, if:
      | -direction of triangle_in is down
      | -user input demands a shift smaller than 1/2 of the period
  note: Shifts triangle_in signal, if:
      | -direction of triangle_in is up
      | -user input demands a shift smaller than 1/2 of the period
  note: Shifts triangle_in signal, if:
      | -direction of triangle_in is up
      | -user input demands a shift larger than 1/2 of the period
  note: Shifts triangle_in signal, if:
      | -direction of triangle_in is down
      | -user input demands a shift larger than 1/2 of the period
  note: Detects, if the triangle_wave is increasing or decreasing
  note: modifies triangle_in signal,
      | if the user demands a shift larger than 1/2 period
  triangle_in : Inport
  triangle_shift : Inport  Port=2
  0 : Constant  Value=0  OutDataTypeStr=boolean  SampleTime=T_FPGA_clk
  Data Type Conversion : DataTypeConversion  OutDataTypeStr=fixdt(1,19,17)
  Data Type Conversion1 : DataTypeConversion  OutDataTypeStr=fixdt(1,20,17)
  Delay1 : Delay  DelayLength=1
  Delay2 : Delay  DelayLength=1
  Gain : Gain  Gain=2  OutDataTypeStr=fixdt(1,20,17)
  Gain1 : Gain  Gain=2  OutDataTypeStr=fixdt(1,20,17)
  Relational Operator1 : RelationalOperator  Operator=<=  OutDataTypeStr=boolean  RndMeth=Nearest
  Relational Operator7 : RelationalOperator  OutDataTypeStr=boolean  RndMeth=Nearest
  Subsystem : Subsystem
  Subsystem1 : Subsystem
  Subsystem2 : Subsystem
  Subsystem3 : Subsystem
  Sum10 : Sum  Inputs=|-+  OutDataTypeStr=fixdt(1,20,17)
  or : Switch  Criteria=u2 > Threshold
  standardized peak of triangle : Constant  OutDataTypeStr=fixdt(0,21,17)  SampleTime=T_FPGA_clk
  sw1 : Switch  Criteria=u2 > Threshold  OutDataTypeStr=fixdt(1,18,16)
  sw2 : Switch  Criteria=u2 > Threshold
  sw3 : Switch  Criteria=u2 > Threshold
  sw4 : Switch  Criteria=u2 > Threshold  Threshold=1  OutDataTypeStr=fixdt(1,20,17)
  triangle_sig : Outport  VectorParamsAs1DForOutWhenUnconnected=off
  wires:
  Subsystem3/1(shifted triangle_in signal) -> sw2/3
  Subsystem2/2(enable_out) -> sw1/2
  Subsystem2/1(shifted triangle_in signal) -> sw1/1
  Subsystem1/1(shifted triangle_in signal) -> sw3/1
  Subsystem1/2(enable_out) -> sw3/2, or/1, or/2
  Subsystem/2(enable_out) -> or/3
  Subsystem/1(shifted triangle_in signal) -> sw3/3
  0/1 -> Subsystem/1(Zero_input), Subsystem1/5(Zero_input), Subsystem2/4(Zero_input)
  Delay1/1 -> Relational Operator1/2
  Relational Operator1/1 -> Subsystem2/5(direction down), Subsystem/5(direction down)  "direction down"
  triangle_in/1 -> Data Type Conversion1/1
  Data Type Conversion/1 -> Gain/1
  sw2/1 -> sw1/3
  Gain1/1 -> Sum10/1
  triangle_shift/1 -> Data Type Conversion/1
  standardized peak of triangle/1 -> Gain1/1, Subsystem1/1(standardized peak of triangle), Subsystem2/3(standardized peak of triangle)  "standardized peak of triangle"
  sw1/1 -> triangle_sig/1
  Sum10/1 -> sw4/1
  Gain/1 -> sw4/2, sw4/3, Subsystem1/3(converted triangle_shift), Subsystem/2(converted triangle_shift), Sum10/2  "converted triangle_shift"
  sw4/1 -> Subsystem2/2(modified triangle_shift), Subsystem1/4(modified triangle_shift), Subsystem/3(modified triangle_shift), Subsystem3/2(modified triangle_shift)  "modified triangle_shift"
  or/1 -> sw2/2
  Relational Operator7/1 -> Subsystem3/3(direction up), Subsystem1/6(direction up)  "direction up"
  sw3/1 -> sw2/1
  Data Type Conversion1/1 -> Relational Operator7/1, Delay2/1, Delay1/1, Relational Operator1/1, Subsystem1/2(triangle_in), Subsystem/4(triangle_in), Subsystem2/1(triangle_in), Subsystem3/1(triangle_in)  "triangle_in"
  Delay2/1 -> Relational Operator7/2

== system gm_IP_Core_SS_Switch_and_PWM/PWM_and_Switching_Signal_Control/GenPWM/Triangle shift/Subsystem ==
  Zero_input : Inport  OutDataTypeStr=boolean  PortDimensions=1  SampleTime=1e-08
  converted triangle_shift : Inport  Port=2  OutDataTypeStr=fixdt(1, 20, 17)  PortDimensions=1  SampleTime=1e-08
  modified triangle_shift : Inport  Port=3  OutDataTypeStr=fixdt(1, 20, 17)  PortDimensions=1  SampleTime=1e-08
  triangle_in : Inport  Port=4  OutDataTypeStr=fixdt(1, 20, 17)  PortDimensions=1  SampleTime=1e-08
  direction down : Inport  Port=5  OutDataTypeStr=boolean  PortDimensions=1  SampleTime=1e-08
  Relational Operator11 : RelationalOperator  Operator=<=  OutDataTypeStr=boolean  SampleTime=1e-08  RndMeth=Nearest
  Sum8 : Sum  Inputs=+-  AccumDataTypeStr=fixdt(1, 21, 17)  OutDataTypeStr=fixdt(1, 21, 17)  SampleTime=1e-08
  Unary Minus : UnaryMinus  SampleTime=1e-08
  and2_1 : Switch  Criteria=u2 > Threshold  Threshold=double(0)  OutDataTypeStr=boolean  SampleTime=1e-08
  and2_2 : Switch  Criteria=u2 > Threshold  Threshold=double(0)  OutDataTypeStr=boolean  SampleTime=1e-08
  delayMatch : Delay  DelayLength=double(1)  InitialCondition=0  SampleTime=1e-08
  delayMatch1 : Delay  DelayLength=double(1)  InitialCondition=0  SampleTime=1e-08
  shifted triangle_in signal : Outport  SampleTime=1e-08
  enable_out : Outport  Port=2  SampleTime=1e-08
  wires:
  delayMatch/1 -> and2_1/3
  Relational Operator11/1 -> and2_1/2
  Sum8/1 -> shifted triangle_in signal/1
  Unary Minus/1 -> Sum8/1, Relational Operator11/2
  and2_1/1 -> and2_2/1
  and2_2/1 -> enable_out/1
  Zero_input/1 -> delayMatch1/1, delayMatch/1
  converted triangle_shift/1 -> and2_1/1
  modified triangle_shift/1 -> Unary Minus/1
  triangle_in/1 -> Sum8/2, Relational Operator11/1
  direction down/1 -> and2_2/2
  delayMatch1/1 -> and2_2/3

== system gm_IP_Core_SS_Switch_and_PWM/PWM_and_Switching_Signal_Control/GenPWM/Triangle shift/Subsystem1 ==
  standardized peak of triangle : Inport  OutDataTypeStr=fixdt(0, 21, 17)  PortDimensions=1  SampleTime=1e-08
  triangle_in : Inport  Port=2  OutDataTypeStr=fixdt(1, 20, 17)  PortDimensions=1  SampleTime=1e-08
  converted triangle_shift : Inport  Port=3  OutDataTypeStr=fixdt(1, 20, 17)  PortDimensions=1  SampleTime=1e-08
  modified triangle_shift : Inport  Port=4  OutDataTypeStr=fixdt(1, 20, 17)  PortDimensions=1  SampleTime=1e-08
  Zero_input : Inport  Port=5  OutDataTypeStr=boolean  PortDimensions=1  SampleTime=1e-08
  direction up : Inport  Port=6  OutDataTypeStr=boolean  PortDimensions=1  SampleTime=1e-08
  Relational Operator2 : RelationalOperator  OutDataTypeStr=boolean  SampleTime=1e-08  RndMeth=Nearest
  Sum11_stage2 : Sum  AccumDataTypeStr=fixdt(1, 24, 17)  OutDataTypeStr=fixdt(1, 24, 17)  SampleTime=1e-08
  Sum11_stage3 : Sum  Inputs=+-  AccumDataTypeStr=fixdt(1, 24, 17)  OutDataTypeStr=fixdt(1, 21, 17)  SampleTime=1e-08
  Sum6 : Sum  AccumDataTypeStr=fixdt(1, 23, 17)  OutDataTypeStr=fixdt(1, 23, 17)  SampleTime=1e-08
  and1_1 : Switch  Criteria=u2 > Threshold  Threshold=double(0)  OutDataTypeStr=boolean  SampleTime=1e-08
  and1_2 : Switch  Criteria=u2 > Threshold  Threshold=double(0)  OutDataTypeStr=boolean  SampleTime=1e-08
  delayMatch{,1..3} (4 alike) : Delay  DelayLength=double(1)  InitialCondition=0  SampleTime=1e-08
  shifted triangle_in signal : Outport  SampleTime=1e-08
  enable_out : Outport  Port=2  SampleTime=1e-08
  wires:
  delayMatch/1 -> Sum6/2
  delayMatch2/1 -> and1_1/3
  Relational Operator2/1 -> and1_1/2
  Sum11_stage3/1 -> shifted triangle_in signal/1
  Sum6/1 -> Sum11_stage2/2, Relational Operator2/2
  and1_1/1 -> and1_2/1
  and1_2/1 -> enable_out/1
  Sum11_stage2/1 -> Sum11_stage3/1
  standardized peak of triangle/1 -> delayMatch1/1, delayMatch/1
  triangle_in/1 -> Sum11_stage3/2, Relational Operator2/1
  converted triangle_shift/1 -> and1_1/1
  modified triangle_shift/1 -> Sum6/1
  Zero_input/1 -> delayMatch3/1, delayMatch2/1
  direction up/1 -> and1_2/2
  delayMatch1/1 -> Sum11_stage2/1
  delayMatch3/1 -> and1_2/3

== system gm_IP_Core_SS_Switch_and_PWM/PWM_and_Switching_Signal_Control/GenPWM/Triangle shift/Subsystem2 ==
  triangle_in : Inport  OutDataTypeStr=fixdt(1, 20, 17)  PortDimensions=1  SampleTime=1e-08
  modified triangle_shift : Inport  Port=2  OutDataTypeStr=fixdt(1, 20, 17)  PortDimensions=1  SampleTime=1e-08
  standardized peak of triangle : Inport  Port=3  OutDataTypeStr=fixdt(0, 21, 17)  PortDimensions=1  SampleTime=1e-08
  Zero_input : Inport  Port=4  OutDataTypeStr=boolean  PortDimensions=1  SampleTime=1e-08
  direction down : Inport  Port=5  OutDataTypeStr=boolean  PortDimensions=1  SampleTime=1e-08
  Relational Operator9 : RelationalOperator  OutDataTypeStr=boolean  SampleTime=1e-08  RndMeth=Nearest
  Sum1 : Sum  Inputs=+-  AccumDataTypeStr=fixdt(1, 23, 17)  OutDataTypeStr=fixdt(1, 23, 17)  SampleTime=1e-08
  Sum5_stage2 : Sum  AccumDataTypeStr=fixdt(1, 24, 17)  OutDataTypeStr=fixdt(1, 24, 17)  SampleTime=1e-08
  Sum5_stage3 : Sum  Inputs=+-  AccumDataTypeStr=fixdt(1, 24, 17)  OutDataTypeStr=fixdt(1, 21, 17)  SampleTime=1e-08
  and : Switch  Criteria=u2 > Threshold  Threshold=double(0)  OutDataTypeStr=boolean  SampleTime=1e-08
  delayMatch : Delay  DelayLength=double(1)  InitialCondition=0  SampleTime=1e-08
  delayMatch1 : Delay  DelayLength=double(1)  InitialCondition=0  SampleTime=1e-08
  delayMatch2 : Delay  DelayLength=double(1)  InitialCondition=0  SampleTime=1e-08
  shifted triangle_in signal : Outport  SampleTime=1e-08
  enable_out : Outport  Port=2  SampleTime=1e-08
  wires:
  delayMatch/1 -> Sum1/1
  delayMatch2/1 -> and/3
  Relational Operator9/1 -> and/1
  Sum1/1 -> Sum5_stage2/1, Relational Operator9/2
  Sum5_stage3/1 -> shifted triangle_in signal/1
  and/1 -> enable_out/1
  Sum5_stage2/1 -> Sum5_stage3/1
  triangle_in/1 -> Sum5_stage3/2, Relational Operator9/1
  modified triangle_shift/1 -> Sum1/2
  standardized peak of triangle/1 -> delayMatch1/1, delayMatch/1
  Zero_input/1 -> delayMatch2/1
  direction down/1 -> and/2
  delayMatch1/1 -> Sum5_stage2/2

== system gm_IP_Core_SS_Switch_and_PWM/PWM_and_Switching_Signal_Control/GenPWM/Triangle shift/Subsystem3 ==
  triangle_in : Inport  OutDataTypeStr=fixdt(1, 20, 17)  PortDimensions=1  SampleTime=1e-08
  modified triangle_shift : Inport  Port=2  OutDataTypeStr=fixdt(1, 20, 17)  PortDimensions=1  SampleTime=1e-08
  direction up : Inport  Port=3  OutDataTypeStr=boolean  PortDimensions=1  SampleTime=1e-08
  Relational Operator6 : RelationalOperator  Operator=<=  OutDataTypeStr=boolean  SampleTime=1e-08  RndMeth=Nearest
  Sum2 : Sum  Inputs=+-  AccumDataTypeStr=fixdt(1, 21, 17)  OutDataTypeStr=fixdt(1, 21, 17)  SampleTime=1e-08
  Sum3 : Sum  Inputs=+-  AccumDataTypeStr=fixdt(1, 21, 17)  OutDataTypeStr=fixdt(1, 21, 17)  SampleTime=1e-08
  Sum4 : Sum  AccumDataTypeStr=fixdt(1, 21, 17)  OutDataTypeStr=fixdt(1, 21, 17)  SampleTime=1e-08
  Switch3 : Switch  Criteria=u2 > Threshold  Threshold=double(0)  OutDataTypeStr=fixdt(1, 21, 17)  SampleTime=1e-08
  sw : Switch  Criteria=u2 > Threshold  Threshold=double(0)  OutDataTypeStr=fixdt(1, 21, 17)  SampleTime=1e-08
  shifted triangle_in signal : Outport  SampleTime=1e-08
  wires:
  Relational Operator6/1 -> Switch3/2
  Sum2/1 -> Switch3/1
  Sum3/1 -> Switch3/3
  Sum4/1 -> sw/3
  Switch3/1 -> sw/1
  sw/1 -> shifted triangle_in signal/1
  triangle_in/1 -> Sum4/2, Sum3/1, Sum2/2, Relational Operator6/1
  modified triangle_shift/1 -> Sum4/1, Sum3/2, Sum2/1, Relational Operator6/2
  direction up/1 -> sw/2

== system gm_IP_Core_SS_Switch_and_PWM/PWM_and_Switching_Signal_Control/GenPWM/Triangle shift1/Subsystem ==
  Zero_input : Inport  OutDataTypeStr=boolean  PortDimensions=1  SampleTime=1e-08
  converted triangle_shift : Inport  Port=2  OutDataTypeStr=fixdt(1, 20, 17)  PortDimensions=1  SampleTime=1e-08
  modified triangle_shift : Inport  Port=3  OutDataTypeStr=fixdt(1, 20, 17)  PortDimensions=1  SampleTime=1e-08
  triangle_in : Inport  Port=4  OutDataTypeStr=fixdt(1, 20, 17)  PortDimensions=1  SampleTime=1e-08
  direction down : Inport  Port=5  OutDataTypeStr=boolean  PortDimensions=1  SampleTime=1e-08
  Relational Operator11 : RelationalOperator  Operator=<=  OutDataTypeStr=boolean  SampleTime=1e-08  RndMeth=Nearest
  Sum8 : Sum  Inputs=+-  AccumDataTypeStr=fixdt(1, 21, 17)  OutDataTypeStr=fixdt(1, 21, 17)  SampleTime=1e-08
  Unary Minus : UnaryMinus  SampleTime=1e-08
  and2_1 : Switch  Criteria=u2 > Threshold  Threshold=double(0)  OutDataTypeStr=boolean  SampleTime=1e-08
  and2_2 : Switch  Criteria=u2 > Threshold  Threshold=double(0)  OutDataTypeStr=boolean  SampleTime=1e-08
  delayMatch : Delay  DelayLength=double(1)  InitialCondition=0  SampleTime=1e-08
  delayMatch1 : Delay  DelayLength=double(1)  InitialCondition=0  SampleTime=1e-08
  shifted triangle_in signal : Outport  SampleTime=1e-08
  enable_out : Outport  Port=2  SampleTime=1e-08
  wires:
  delayMatch/1 -> and2_1/3
  Relational Operator11/1 -> and2_1/2
  Sum8/1 -> shifted triangle_in signal/1
  Unary Minus/1 -> Sum8/1, Relational Operator11/2
  and2_1/1 -> and2_2/1
  and2_2/1 -> enable_out/1
  Zero_input/1 -> delayMatch1/1, delayMatch/1
  converted triangle_shift/1 -> and2_1/1
  modified triangle_shift/1 -> Unary Minus/1
  triangle_in/1 -> Sum8/2, Relational Operator11/1
  direction down/1 -> and2_2/2
  delayMatch1/1 -> and2_2/3
